simulink model "Displays_ARES_Sim"  (R2019b)
settings: Solver=FixedStepAuto  StartTime=0  StopTime=500  RelTol=1e-3  EnableMultiTasking=on
values from neighbouring files (symbols this model uses):
  Avail_Mode = 2    [Init_Vars_ARES_Sim.m]    (also in Init_Vars_ARES_Sim_SR.m = 0; Init_Vars_ARES_Sim_SR_Michael.m = 0)
  quad_s = 1    [Init_Vars_ARES_Sim.m]    (also in Init_Vars_ARES_Sim_SR.m; Init_Vars_ARES_Sim_SR_Michael.m)
  xLP0 = x0    (= 12000)    [Init_Vars_ARES_Sim.m]    (also in Init_Vars_ARES_Sim_SR.m; Init_Vars_ARES_Sim_SR_Michael.m)
  yLP0 = y0 + 1350    (= 13350)    [Init_Vars_ARES_Sim.m]    (also in Init_Vars_ARES_Sim_SR.m = 10950; Init_Vars_ARES_Sim_SR_Michael.m = 10950)
undefined symbols (not defined in the file or in its folder): LPs, var
libraries: vrlib x37, simulink x5, visionsources x3, simulink_extras x1, aerolibanimutils x1
(part 1 of 2)
settings Model: PacingRate=1.200000  Creator=DreamChaser  LastModifiedBy=ARES
settings SolverCC: AutoInsertRateTranBlk=on
settings DataIOCC: ReturnWorkspaceOutputs=off
settings DebuggingCC: MultiTaskDSMMsg=none  ArithmeticOperatorsInVariantConditions=warning
settings SFSimCC: SimUseLocalCustomCode=off  CustomCodeUndefinedFunction=UseInterfaceOnly
settings RTWCC: RTWUseLocalCustomCode=off
settings CodeAppCC: StateflowObjectComments=on

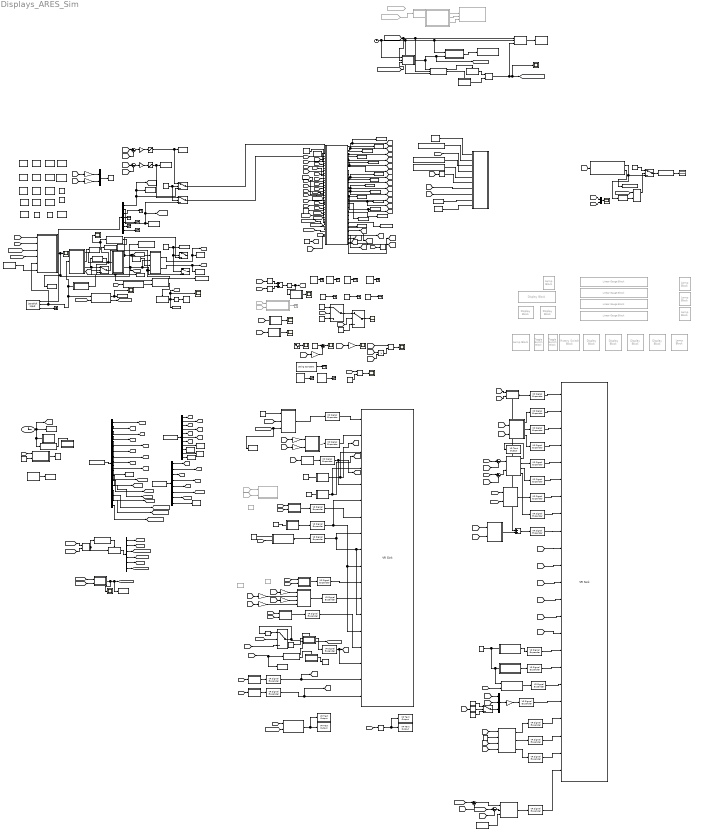
== system Displays_ARES_Sim ==
  note: Stop simulation at LP height
  note: Assure that you run initvars script
  note: Clock and Stop Condition
  note: Define Vehicle Dynamics
  note: Memory blocks intialization
  note: Input variables from Matlab
  note: Failure Modes
  note: SYSTEM DISPLAY
  note: Cache
  note: Groundspeed
  note: Heading
  note: Clearing
  note: Lunar Bat
  note: LMP Bat 2
  note: LMP Bat 1
  note: DECENT POWER
  note: COMS STATUS
  note: LANDING CONDITIONS
  note: Speed
  note: Roll
  note: Pitch
  note: LIDAR CONTROL
  note: Active
  note: Main
  note: Gain
  note: Aux
  note: Tertiary Flight Display
  note: Pitch & Roll Alarms
  note: LIDAR CONTROL
  note: COMS STATUS
  note: DECENT POWER
  note: SYSTEM DISPLAY
  note: Thrust
  note: Fuel Temp
  note: Fuel
      | Press
  note: T/W
  note: Lunar Contact
  note: Background Translation
  note: Altitude Marker
  note: Landing Site Bar
  note: Fuel bar
  note: Subject Roll Triangle
  note: Primary Flight Display (Design done in the VRSink block: assure the VRsink is open)
  note: Gudiance Cues Translation
  note: Pitch Translation Bar
  note: Background Rotation
  note: Pitch Rotation Bars
  note: Terminal Descent Bar
  note: Roll Guidance Triangle
  note: Pitch Rotation
  note: Pitch Text
  note: Autopilot 0.1
  note: HSI - Horizontal Situation Indicator
  note: Embedded Tasks
  note: Redesignation of landing sites
      | (Improvements need to be
      | made here for run speed)
  note: Workload Assessment (B&E test)
  "  2" : ToWorkspace  VariableName=abort_press  SaveFormat=Timeseries  SampleTime=-1
  "  3" : ToWorkspace  VariableName=valid_abort  SaveFormat=Timeseries  SampleTime=-1
  " 2" : ToWorkspace  VariableName=fail_detection_time  SaveFormat=Timeseries  SampleTime=-1
  " 3" : ToWorkspace  VariableName=fail_detection  SaveFormat=Timeseries  SampleTime=-1
  ASCII to String1 : ASCIIToString
  AUTO Mode Select1 : MATLAB Function  TreatAsAtomicUnit=on
  AUTO Mode Select3 : MATLAB Function  TreatAsAtomicUnit=on
  Abort_Value_Func1 : MATLAB Function  TreatAsAtomicUnit=on
  Active LIDAR : Scope
  Add : Sum
  Add1 : Sum
  Alt Triangle Pts : MATLAB Function  TreatAsAtomicUnit=on
  Aux : Terminator
  B&E function1 : MATLAB Function  TreatAsAtomicUnit=on
  B&E test1 : Display
  Background Translation : MATLAB Function  TreatAsAtomicUnit=on
  Clock : Clock
  Clock1 : Clock
  Compare To Constant : simulink/Logic and Bit Operations/Compare To Constant  relop=<=  const=250  OutDataTypeStr=boolean
  Compare To Constant1 : simulink/Logic and Bit Operations/Compare To Constant  relop=<=  const=250  OutDataTypeStr=boolean
  Constant1 : Constant  Value=Avail_Mode
  Constant11 : Constant  Value=Avail_Mode
  Constant12 : Constant  Value=3
  Constant13 : Constant  Value=100
  Constant14 : Constant  Value=260  SampleTime=-1
  Constant15 : Constant  Value=0
  Constant16 : Constant  Value=8  OutDataTypeStr=uint8
  Constant2 : Constant  Value=quad_s
  Constant22 : Constant  Value=1000
  Constant23 : Constant  Value=1.1
  Constant5 : Constant
  Constant6 : Constant
  Constant7 : Constant  Value=0
  Constant8 : Constant
  Constant9 : Constant  Value=3
  "Contact LIght " : Scope
  Data Store Memory : DataStoreMemory  DataStoreName=xLPPos  ReadBeforeWriteMsg=warning  WriteAfterWriteMsg=warning  WriteAfterReadMsg=warning  ShowAdditionalParam=off
  Data Store Memory1 : DataStoreMemory  DataStoreName=yLPPos  ReadBeforeWriteMsg=warning  WriteAfterWriteMsg=warning  WriteAfterReadMsg=warning  ShowAdditionalParam=off
  Data Store Memory10 : DataStoreMemory  DataStoreName=hTD  ReadBeforeWriteMsg=warning  WriteAfterWriteMsg=warning  WriteAfterReadMsg=warning  ShowAdditionalParam=off
  Data Store Memory11 : DataStoreMemory  DataStoreName=hLP  ReadBeforeWriteMsg=warning  WriteAfterWriteMsg=warning  WriteAfterReadMsg=warning  ShowAdditionalParam=off
  Data Store Memory12 : DataStoreMemory  DataStoreName=mp_guess  ReadBeforeWriteMsg=warning  WriteAfterWriteMsg=warning  WriteAfterReadMsg=warning  ShowAdditionalParam=off
  Data Store Memory13 : DataStoreMemory  DataStoreName=fail_type  ReadBeforeWriteMsg=warning  WriteAfterWriteMsg=warning  WriteAfterReadMsg=warning  ShowAdditionalParam=off
  Data Store Memory14 : DataStoreMemory  DataStoreName=quad_s  ReadBeforeWriteMsg=warning  WriteAfterWriteMsg=warning  WriteAfterReadMsg=warning  ShowAdditionalParam=off
  Data Store Memory17 : DataStoreMemory  DataStoreName=Mode  ReadBeforeWriteMsg=warning  WriteAfterWriteMsg=warning  WriteAfterReadMsg=warning  ShowAdditionalParam=off
  Data Store Memory19 : DataStoreMemory  DataStoreName=x_delta  ReadBeforeWriteMsg=warning  WriteAfterWriteMsg=warning  WriteAfterReadMsg=warning  ShowAdditionalParam=off
  Data Store Memory2 : DataStoreMemory  DataStoreName=xLPNeg  ReadBeforeWriteMsg=warning  WriteAfterWriteMsg=warning  WriteAfterReadMsg=warning  ShowAdditionalParam=off
  Data Store Memory20 : DataStoreMemory  DataStoreName=y_delta  ReadBeforeWriteMsg=warning  WriteAfterWriteMsg=warning  WriteAfterReadMsg=warning  ShowAdditionalParam=off
  Data Store Memory3 : DataStoreMemory  DataStoreName=yLPNeg  ReadBeforeWriteMsg=warning  WriteAfterWriteMsg=warning  WriteAfterReadMsg=warning  ShowAdditionalParam=off
  Data Store Memory4 : DataStoreMemory  DataStoreName=yLPNew  ReadBeforeWriteMsg=warning  WriteAfterWriteMsg=warning  WriteAfterReadMsg=warning  ShowAdditionalParam=off
  Data Store Memory5 : DataStoreMemory  DataStoreName=xLPNew  ReadBeforeWriteMsg=warning  WriteAfterWriteMsg=warning  WriteAfterReadMsg=warning  ShowAdditionalParam=off
  Data Store Memory6 : DataStoreMemory  DataStoreName=intervalPos  ReadBeforeWriteMsg=warning  WriteAfterWriteMsg=warning  WriteAfterReadMsg=warning  ShowAdditionalParam=off
  Data Store Memory7 : DataStoreMemory  DataStoreName=intervalNeg  ReadBeforeWriteMsg=warning  WriteAfterWriteMsg=warning  WriteAfterReadMsg=warning  ShowAdditionalParam=off
  Data Store Memory8 : DataStoreMemory  DataStoreName=interval  ReadBeforeWriteMsg=warning  WriteAfterWriteMsg=warning  WriteAfterReadMsg=warning  ShowAdditionalParam=off
  Data Store Memory9 : DataStoreMemory  DataStoreName=R0val  ReadBeforeWriteMsg=warning  WriteAfterWriteMsg=warning  WriteAfterReadMsg=warning  InitialValue=1e-12  ShowAdditionalParam=off  OutDataTypeStr=double
  Data Store Read : DataStoreRead  DataStoreName=xLPNew  SampleTime=0.1
  Data Store Read1 : DataStoreRead  DataStoreName=yLPNew  SampleTime=0.1
  Data Store Read10 : DataStoreRead  DataStoreName=hLP
  Data Store Read11 : DataStoreRead  DataStoreName=hTD
  Data Store Read12 : DataStoreRead  DataStoreName=hLP  SampleTime=0.1
  Data Store Read13 : DataStoreRead  DataStoreName=hLP  SampleTime=0.1
  Data Store Read18 : DataStoreRead  DataStoreName=hLP  SampleTime=0.1
  Data Store Read2 : DataStoreRead  DataStoreName=xLPNew
  Data Store Read21 : DataStoreRead  DataStoreName=R0val  SampleTime=0.1
  Data Store Read3 : DataStoreRead  DataStoreName=yLPNew
  Data Store Read{36..39} (4 alike) : DataStoreRead  DataStoreName=Mode
  Data Store Read6 : DataStoreRead  DataStoreName=interval
  Data Store Write12 : DataStoreWrite  DataStoreName=hTD  SampleTime=0.1
  Data Store Write13 : DataStoreWrite  DataStoreName=hLP  SampleTime=0.1
  Data Store Write14 : DataStoreWrite  DataStoreName=xLPNew  SampleTime=0.1
  Data Store Write15 : DataStoreWrite  DataStoreName=yLPNew  SampleTime=0.1
  Data Store Write20 : DataStoreWrite  DataStoreName=interval  SampleTime=0.1
  Data Store Write22 : DataStoreWrite  DataStoreName=yLPNew  SampleTime=0.1
  Data Store Write3 : DataStoreWrite  DataStoreName=Mode
  Data Store Write6 : DataStoreWrite  DataStoreName=xLPNew  SampleTime=0.1
  Data Store Write8 : DataStoreWrite  DataStoreName=R0val  SampleTime=0.1
  Define Buttons LPs1 : MATLAB Function  TreatAsAtomicUnit=on
  Delay One Step : Delay  DelayLengthSource=Input port  DelayLength=1  DelayLengthUpperLimit=3000
      settings: InputPortMap=u0,p1
  Delay1 : Delay  DelayLength=6  InitialCondition=0
  Demux : Demux  Outputs=7
  Demux2 : Demux  Outputs=6
  Demux3 : Demux  Outputs=8
  Demux6 : Demux  Outputs=11
  Demux7 : Demux  Outputs=18
  Descent Rate output : ToWorkspace  VariableName=hdot  SaveFormat=Timeseries  SampleTime=-1
  Designated Landing : MATLAB Function  TreatAsAtomicUnit=on
  Designated hTD : MATLAB Function  TreatAsAtomicUnit=on
  Detect Change5 : simulink/Logic and Bit Operations/Detect Change  vinit=0  OutDataTypeStr=boolean
  Detect Increase1 : simulink/Logic and Bit Operations/Detect Increase  vinit=0.0  OutDataTypeStr=boolean
  Detect Increase4 : simulink/Logic and Bit Operations/Detect Increase  vinit=0.0  OutDataTypeStr=boolean
  Display{1..7} (7 alike) : DisplayBlock  Commented=on  LabelPosition=Hide  Format=short  Transparency=1
  Divide : Product  Inputs=*/
  From Workspace1 : FromWorkspace  VariableName=constant_vars  SampleTime=0
  From Workspace2 : FromWorkspace  VariableName=Initial_conditions  SampleTime=0
  From Workspace5 : FromWorkspace  VariableName=input_vars  SampleTime=0
  From135 : From  Commented=on  GotoTag=fuel
  From136 : From  Commented=on  GotoTag=mdot
  From27 : From  Commented=on  GotoTag=buzz_time_1
  From29 : From  Commented=on  GotoTag=buzz_time_2
  From95 : From  Commented=on  GotoTag=VE
  From96 : From  Commented=on  GotoTag=VN
  Fuel Press : Scope
  Fuel Temp : Scope
  Gain{,2..4,6..7} (6 alike) : Gain  Gain=0.1
  Gain1 : Gain  Gain=.1
  Gain10 : Gain  Gain=20/6000
  Gain11 : Gain  Gain=1/3
  Gain12 : Gain  Gain=1/3
  Gain13 : Gain  Gain=-0.01
  Gain5 : Gain  Gain=.1
  Gain9 : Gain  Gain=100/6000
  GreaterThan3 : RelationalOperator  Operator=<=  OutDataTypeStr=boolean  RndMeth=Simplest
  Groundspeed : MATLAB Function  TreatAsAtomicUnit=on
  Guidance Cross : MATLAB Function  TreatAsAtomicUnit=on
  Guidance Triangle : MATLAB Function  TreatAsAtomicUnit=on
  HSD_model : ModelReference  ModelNameDialog=HSD_model  SimulationMode=Normal  ModelReferenceVersion=1.1662
  HSI_Acc1 : MATLAB Function  TreatAsAtomicUnit=on
  HSI_Ball : MATLAB Function  TreatAsAtomicUnit=on
  HSI_LP : MATLAB Function  TreatAsAtomicUnit=on
  HSI_VG : MATLAB Function  TreatAsAtomicUnit=on
  HSI_Vec : MATLAB Function  TreatAsAtomicUnit=on
  Heading : Terminator  Commented=on
  IPC Mode Select2 : MATLAB Function  TreatAsAtomicUnit=on
  If : If  ElseIfExpressions=u1<0  ShowElse=off
  If Action Subsystem : Subsystem  TreatAsAtomicUnit=on
  If Action Subsystem1 : Subsystem  TreatAsAtomicUnit=on
  If Action Subsystem2 : Subsystem  TreatAsAtomicUnit=on
  If Action Subsystem3 : Subsystem  TreatAsAtomicUnit=on
  If Action Subsystem5 : Subsystem  TreatAsAtomicUnit=on
  If Action Subsystem6 : Subsystem  TreatAsAtomicUnit=on
  If Action Subsystem7 : Subsystem  TreatAsAtomicUnit=on
  If Action Subsystem8 : Subsystem  TreatAsAtomicUnit=on
  If Action Subsystem9 : Subsystem  TreatAsAtomicUnit=on
  If1 : If  NumInputs=3  IfExpression=u1==1  ElseIfExpressions=u2==u3
  If2 : If  IfExpression=u1 ~= 0  ShowElse=off
  If4 : If  ShowElse=off
  If5 : If  IfExpression=u1 ~= 0  ShowElse=off
  If6 : If  IfExpression=u1 < 0.0003  ShowElse=off
  If9 : If  NumInputs=2  IfExpression=u1 ==1 & u2 ==1  ShowElse=off
  Image From File7 : visionsources/Image From File  Tag=vipblks_nd  FileName=C:\Users\ARES\Documents\ARES Simulation SR\Graphics\Abort_Photo_V1.jpg  Ts=-1  imagePorts=One multidimensional signal  OutPortLabels=R|G|B  ImageDataType=int32  sdImageDataType=uint(8)  Signed=on  WordLength=16  FractionLengthMode=User-defined  FractionLength=15
      settings: SourceProductName=Computer Vision Toolbox
  Image From File8 : visionsources/Image From File  Tag=vipblks_nd  FileName=C:\Users\ARES\Documents\ARES Simulation SR\ALD_Map_Hazzards.png  Ts=-1  imagePorts=One multidimensional signal  OutPortLabels=R|G|B  ImageDataType=int32  sdImageDataType=uint(8)  Signed=on  WordLength=16  FractionLengthMode=User-defined  FractionLength=15
      settings: SourceProductName=Computer Vision Toolbox
  Image From File9 : visionsources/Image From File  Tag=vipblks_nd  FileName=C:\Users\ARES\Documents\ARES Simulation SR\ALD_Map_No_Hazzards.png  Ts=-1  imagePorts=One multidimensional signal  OutPortLabels=R|G|B  ImageDataType=int32  sdImageDataType=uint(8)  Signed=on  WordLength=16  FractionLengthMode=User-defined  FractionLength=15
      settings: SourceProductName=Computer Vision Toolbox
  Joystick Input2 : vrlib/Joystick Input  joyid=1  adjustports=on  forcefeed=off
      settings: SourceProductBaseCode=VR
  LMP 1 : Terminator
  LMP 2 : Terminator
  Lamp{,1..5} (6 alike) : LampBlock  Commented=on  LabelPosition=Hide
  Lidar Gain : Terminator
  Linear Gauge : LinearGaugeBlock  Commented=on  LabelPosition=Hide  TickInterval=20
  Linear Gauge1 : LinearGaugeBlock  Commented=on  LabelPosition=Hide  ScaleMin=40  TickInterval=10
  Linear Gauge2 : LinearGaugeBlock  Commented=on  LabelPosition=Hide  ScaleMax=6  TickInterval=1
  Linear Gauge3 : LinearGaugeBlock  Commented=on  LabelPosition=Hide  ScaleMax=300  TickInterval=50
  Lunar Bat : Terminator
  MA : Terminator
  MATLAB Function : MATLAB Function  Commented=on  TreatAsAtomicUnit=on
  MATLAB Function1 : MATLAB Function  TreatAsAtomicUnit=on
  MATLAB Function10 : MATLAB Function  Commented=on  TreatAsAtomicUnit=on
  MATLAB Function11 : MATLAB Function  TreatAsAtomicUnit=on
  MATLAB Function12 : MATLAB Function  TreatAsAtomicUnit=on
  MATLAB Function13 : MATLAB Function  TreatAsAtomicUnit=on
  MATLAB Function14 : MATLAB Function  TreatAsAtomicUnit=on
  MATLAB Function15 : MATLAB Function  TreatAsAtomicUnit=on
  MATLAB Function16 : MATLAB Function  TreatAsAtomicUnit=on
  MATLAB Function17 : MATLAB Function  TreatAsAtomicUnit=on
  MATLAB Function18 : MATLAB Function  TreatAsAtomicUnit=on
  MATLAB Function2 : MATLAB Function  TreatAsAtomicUnit=on
  MATLAB Function3 : MATLAB Function  Commented=on  TreatAsAtomicUnit=on
  MATLAB Function4 : MATLAB Function  Commented=on  TreatAsAtomicUnit=on
  MATLAB Function5 : MATLAB Function  TreatAsAtomicUnit=on
  MATLAB Function6 : MATLAB Function  TreatAsAtomicUnit=on
  MATLAB Function7 : MATLAB Function  Commented=on  TreatAsAtomicUnit=on
  MATLAB Function8 : MATLAB Function  TreatAsAtomicUnit=on
  MATLAB Function9 : MATLAB Function  TreatAsAtomicUnit=on
  Main : Terminator
  Memory : Memory
  Merge : Merge
  Mux : Mux  Inputs=2
  Mux3 : Mux  Inputs=3
  Mux4 : Mux  Inputs=2
  Overpitch Scope : Scope
  Overroll Scope : Scope
  Overspeed Scope : Scope
  Pitch & Roll1 : Scope
  Pitch Translation Bars : MATLAB Function  TreatAsAtomicUnit=on
  Pitch TranslationText : MATLAB Function  TreatAsAtomicUnit=on
  Product : Product
  Pulse Generator : DiscretePulseGenerator  PulseType=Time based  Period=1/6  PulseWidth=50
  RCAH Mode Select1 : MATLAB Function  TreatAsAtomicUnit=on
  Roll Triangle : MATLAB Function  TreatAsAtomicUnit=on
  Rotary Switch : RotarySwitchBlock  Commented=on  LabelPosition=Hide
      settings: Values={{'Off', 'Low', 'Medium', 'High'}, [0 1 2 3]}
  Rotations : MATLAB Function  TreatAsAtomicUnit=on
  Round : Rounding  Operator=round
  S-R Flip-Flop1 : simulink_extras/Flip Flops/S-R Flip-Flop  initial_condition=0
  Saturation : Saturate  UpperLimit=1  LowerLimit=-1
  Saturation1 : Saturate  UpperLimit=1  LowerLimit=-1
  Scope{,1..5} (6 alike) : Scope
  Secondary Workload : MATLAB Function  TreatAsAtomicUnit=on
  Simulation Pace : aerolibanimutils/Simulation Pace  SimulationPace=1  SleepMode=MATLAB Thread  OutputPaceError=off  SampleTime=1/30
  Sine Wave : Sin  Amplitude=2  Bias=70  Frequency=2*pi/120  SampleTime=0
  Sqrt : Sqrt  SaturateOnIntegerOverflow=on
  Square : Math  Operator=square  SignedPower=off  SaturateOnIntegerOverflow=on
  Square1 : Math  Operator=square  SignedPower=off  SaturateOnIntegerOverflow=on
  Stop Simulation2 : Stop
  Stop Simulation3 : Stop
  Stop Simulation4 : Stop
  String Constant1 : StringConstant  String="\"29 V\""
  String Constant2 : StringConstant  String="\"30 V\""
  String Constant3 : StringConstant  String="\"32 V\""
  String Constant4 : StringConstant  String="\"AQ\""
  String Constant5 : StringConstant  String="\"MASTER ALARM\""
  String Constant6 : StringConstant  String="\"TEMP\""
  String Constant7 : StringConstant  String="\"NO ATT\""
  Subsystem1 : Subsystem
  Sum{,1..2,4..7} (7 alike) : Sum  Inputs=|+-
  Switch{,7..8,10..12} (6 alike) : Switch  Criteria=u2 > Threshold
  Switch2 : Switch  Criteria=u2 > Threshold  Threshold=1
  Switch3 : Switch  Criteria=u2 > Threshold  Threshold=250
  Switch4 : Switch  Criteria=u2 > Threshold  Threshold=225
  Switch5 : Switch  Criteria=u2 > Threshold  Threshold=1
  T/W : Scope
  "TA " : Terminator
  TA 1 : Terminator
  Terminator{,1..4,6} (6 alike) : Terminator
  Thrust : Scope
  To Workspace : ToWorkspace  VariableName=R  SaveFormat=Timeseries  SampleTime=-1
  To Workspace1 : ToWorkspace  VariableName=thetaG  SaveFormat=Timeseries  SampleTime=-1
  To Workspace10 : ToWorkspace  VariableName=LP_button  SaveFormat=Timeseries  SampleTime=-1
  To Workspace11 : ToWorkspace  VariableName=IPC_button  SaveFormat=Timeseries  SampleTime=-1
  To Workspace13 : ToWorkspace  VariableName=roll_gain_fail  SaveFormat=Timeseries  SampleTime=-1
  To Workspace14 : ToWorkspace  VariableName=pitch_gain_fail  SaveFormat=Timeseries  SampleTime=-1
  To Workspace15 : ToWorkspace  VariableName=reversal_fail  SaveFormat=Timeseries  SampleTime=-1
  To Workspace16 : ToWorkspace  VariableName=stuck_fail  SaveFormat=Timeseries  SampleTime=-1
  To Workspace17 : ToWorkspace  VariableName=fail_percent  SaveFormat=Timeseries  SampleTime=-1
  To Workspace18 : ToWorkspace  VariableName=RealTime  SampleTime=-1
  To Workspace19 : ToWorkspace  VariableName=fail_roll_triangle  SaveFormat=Timeseries  SampleTime=-1
  To Workspace2 : ToWorkspace  VariableName=phiG  SaveFormat=Timeseries  SampleTime=-1
  To Workspace20 : ToWorkspace  VariableName=fuel_fail_out  SaveFormat=Timeseries  SampleTime=-1
  To Workspace24 : ToWorkspace  VariableName=pitch_comm1  SaveFormat=Timeseries  SampleTime=-1
  To Workspace25 : ToWorkspace  VariableName=roll_comm1  SaveFormat=Timeseries  SampleTime=-1
  To Workspace3 : ToWorkspace  VariableName=Time  SaveFormat=Timeseries  SampleTime=-1
  To Workspace4 : ToWorkspace  VariableName=fuel  SaveFormat=Timeseries  SampleTime=-1
  To Workspace5 : ToWorkspace  VariableName=pitch_comm  SaveFormat=Timeseries  SampleTime=-1
  To Workspace6 : ToWorkspace  VariableName=roll_comm  SaveFormat=Timeseries  SampleTime=-1
  To Workspace7 : ToWorkspace  VariableName=Auditory_TIME_BUTTON  SaveFormat=Timeseries  SampleTime=-1
      settings: Save2DSignal=2-D array (concatenate along first dimension)
  Toggle Switch : ToggleSwitchBlock  Commented=on  LabelPosition=Hide
      settings: Values={{'Off', 'On'}, [0 1]}
  Toggle Switch1 : ToggleSwitchBlock  Commented=on  LabelPosition=Hide
      settings: Values={{'Off', 'On'}, [0 1]}
  Uplink : Terminator
  VE output : ToWorkspace  VariableName=VE  SaveFormat=Timeseries  SampleTime=-1
      settings: Save2DSignal=2-D array (concatenate along first dimension)
  VN output : ToWorkspace  VariableName=VN  SaveFormat=Timeseries  SampleTime=-1
  VN output2 : ToWorkspace  VariableName=Mode  SaveFormat=Timeseries  SampleTime=-1
  VR Signal Expander : vrlib/VR Signal Expander  outwidth=3  outidx=[1,2,3]
      settings: SourceProductName=Simulink 3D Animation  SourceProductBaseCode=VR
  VR Signal Expander1 : vrlib/VR Signal Expander  outwidth=3  outidx=[1,2,3]
      settings: SourceProductName=Simulink 3D Animation  SourceProductBaseCode=VR
  VR Signal Expander10 : vrlib/VR Signal Expander  outwidth=3  outidx=[2]
      settings: SourceProductName=Simulink 3D Animation  SourceProductBaseCode=VR
  VR Signal Expander{5,8,11,23,33..36} (8 alike) : vrlib/VR Signal Expander  outwidth=3  outidx=[1 2 3]
      VR Signal Expander11 settings: SourceProductName=Simulink
      VR Signal Expander23 settings: SourceProductName=Simulink
      VR Signal Expander33 settings: SourceProductName=Simulink
      VR Signal Expander34 settings: SourceProductName=Simulink
      VR Signal Expander35 settings: SourceProductName=Simulink
      VR Signal Expander36 settings: SourceProductName=Simulink
      VR Signal Expander5 settings: SourceProductName=Simulink 3D Animation  SourceProductBaseCode=VR
      VR Signal Expander8 settings: SourceProductName=Simulink 3D Animation  SourceProductBaseCode=VR
  VR Signal Expander{2,6..7,12..13,17,30..32} (9 alike) : vrlib/VR Signal Expander  outwidth=3  outidx=[1 2]
      VR Signal Expander12 settings: SourceProductName=Simulink
      VR Signal Expander13 settings: SourceProductName=Simulink
      VR Signal Expander17 settings: SourceProductName=Simulink
      VR Signal Expander2 settings: SourceProductName=Simulink 3D Animation  SourceProductBaseCode=VR
      VR Signal Expander30 settings: SourceProductName=Simulink
      VR Signal Expander31 settings: SourceProductName=Simulink
      VR Signal Expander32 settings: SourceProductName=Simulink
      VR Signal Expander6 settings: SourceProductName=Simulink 3D Animation  SourceProductBaseCode=VR
      VR Signal Expander7 settings: SourceProductName=Simulink 3D Animation  SourceProductBaseCode=VR
  VR Signal Expander14 : vrlib/VR Signal Expander  outwidth=4  outidx=[4]
      settings: SourceProductName=Simulink
  VR Signal Expander15 : vrlib/VR Signal Expander  outwidth=3  outidx=[2]
      settings: SourceProductName=Simulink
  VR Signal Expander16 : vrlib/VR Signal Expander  outwidth=4  outidx=[4]
      settings: SourceProductName=Simulink
  VR Signal Expander18 : vrlib/VR Signal Expander  outwidth=3  outidx=[3]
      settings: SourceProductName=Simulink
  VR Signal Expander19 : vrlib/VR Signal Expander  outwidth=3  outidx=[3]
      settings: SourceProductName=Simulink
  VR Signal Expander20 : vrlib/VR Signal Expander  outwidth=3  outidx=[3]
      settings: SourceProductName=Simulink
  VR Signal Expander3 : vrlib/VR Signal Expander  outwidth=4  outidx=[3 4]
      settings: SourceProductName=Simulink 3D Animation  SourceProductBaseCode=VR
  VR Signal Expander4 : vrlib/VR Signal Expander  outwidth=3  outidx=[1,2]
      settings: SourceProductName=Simulink 3D Animation  SourceProductBaseCode=VR
  VR Signal Expander9 : vrlib/VR Signal Expander  outwidth=3  outidx=[1,2,3]
      settings: SourceProductName=Simulink 3D Animation  SourceProductBaseCode=VR
  VR Sink : vrlib/VR Sink  InstantiateOnLoad=on  SampleTime=0.1  ViewEnable=on  RemoteChange=off  RemoteView=off  FieldsWritten=Vel_Ball.translation.3.1.1.double#Vel_Vector.rotation.4.1.1.double#Vel_Vector.scale.3.1.1.double#Vel_Vector.translation.3.1.1.double#Guide_Heading_Rot.rotation.4.1.1.double#LP.translation.3.1.1.double#Guidance_Velocity.translation.3.1.1.double#Landing_Point.translation.3.1.1.double#Ship_accel.translation.3.1.1.double#FuelGauge.scale.3.1.1.double#DesignatedLanding.translation.3.1.1.double#DesignatedHTD.translation.3.1.1.double#AltitudeTriangle.translation.3.1.1.double#AltitudeTriangle_0002.translation.3.1.1.double#AltitudeTriangle_0001.translation.3.1.1.double#RCAH_Color.diffuseColor.3.1.1.double#IPC_Color.diffuseColor.3.1.1.double#AUTO_Color.diffuseColor.3.1.1.double#Map.translation.3.1.1.double#Abort.translation.3.1.1.double#Land.translation.3.1.1.double#Fuel_img.translation.3.1.1.double#Original_LP.translation.3.1.1.double  WorldFileName=VRWorlds\hsi.wrl  AutoView=on  VideoDimensions=[]  AllowVariableSize=off  FigureProperties="{'Position', 'Name', 'Viewpoint', 'CameraBound', 'CameraDirection', 'CameraPosition', 'CameraUpVector', 'ZoomFactor', 'Antialiasing', 'Headlight', 'Lighting', 'NavPanel', 'Sound', 'StatusBar', 'Stereo3D', 'Stereo3DCameraOffset', 'Stereo3DHIT', 'ToolBar', 'Textures', 'Transparency', 'Triad', 'Wireframe', 'NavZones', 'NavMode', 'NavSpeed', 'CaptureFileFormat', 'CaptureFileName', 'Record2DCompressMethod', 'Record2DCompressQuality', 'Record2D', 'Record2DFileName', 'Record2DFPS'; [-1.0240000000000000e+03   7.2500000000000000e+02   1.0200000000000000e+03   5.0200000000000000e+02], '', '_untitled_1', 'on', [7.1821279555918119e-02  -7.1914500889074973e-02  -9.9482159624971234e-01], [0.0000000000000000e+00   0.0000000000000000e+00   0.0000000000000000e+00], [3.8829635941558640e-03   9.9740995904225715e-01  -7.1821279555918133e-02], [1.0000000000000000e+00], 'on', 'on', 'on', 'halfbar', 'on', 'on', 'off', [1.0000000149011612e-01], [0.0000000000000000e+00], 'on', 'on', 'on', 'none', 'off', 'off', 'fly', 'normal', 'tif', '%f_anim_%n.tif', 'auto', [7.5000000000000000e+01], 'off', '%f_anim_%n.avi', 'auto'}"
      settings: SourceProductName=Simulink
  VR Sink1 : vrlib/VR Sink  InstantiateOnLoad=on  SampleTime=0.1  ViewEnable=on  RemoteChange=off  RemoteView=off  FieldsWritten=BotTriangle.translation.3.1.1.double#TopTriangle.translation.3.1.1.double#DesignatedLanding.translation.3.1.1.double#DesignatedHTD.translation.3.1.1.double#AltitudeTriangle.translation.3.1.1.double#Rotating.rotation.4.1.1.double#Rotating.translation.3.1.1.double#Right_bar.diffuseColor.3.1.1.double#LeftPitch.diffuseColor.3.1.1.double#PitchText.rotation.4.1.1.double#PitchText.translation.3.1.1.double#Cross.translation.3.1.1.double#Piper.diffuseColor.3.1.1.double#BotBack.rotation.4.1.1.double#BotBack.translation.3.1.1.double#FuelGauge.scale.3.1.1.double#AltitudeTriangle_0001.translation.3.1.1.double#AltitudeTriangle_0002.translation.3.1.1.double  WorldFileName=VRWorlds\VRWorld1.wrl  AutoView=on  VideoDimensions=[]  AllowVariableSize=off  FigureProperties="{'Position', 'Name', 'Viewpoint', 'CameraBound', 'CameraDirection', 'CameraPosition', 'CameraUpVector', 'ZoomFactor', 'Antialiasing', 'Headlight', 'Lighting', 'NavPanel', 'Sound', 'StatusBar', 'Stereo3D', 'Stereo3DCameraOffset', 'Stereo3DHIT', 'ToolBar', 'Textures', 'Transparency', 'Triad', 'Wireframe', 'NavZones', 'NavMode', 'NavSpeed', 'CaptureFileFormat', 'CaptureFileName', 'Record2DCompressMethod', 'Record2DCompressQuality', 'Record2D', 'Record2DFileName', 'Record2DFPS'; [-1.0180000000000000e+03   7.3000000000000000e+01   1.0080000000000000e+03   5.8200000000000000e+02], '', 'View', 'on', [3.1395253498715962e-02  -3.1410752802896694e-02  -9.9901336460835521e-01], [0.0000000000000000e+00   0.0000000000000000e+00   0.0000000000000000e+00], [9.8663539164468286e-04   9.9950656056293863e-01  -3.1395253498715962e-02], [1.0000000000000000e+00], 'on', 'on', 'on', 'halfbar', 'on', 'off', 'off', [1.0000000149011612e-01], [0.0000000000000000e+00], 'off', 'on', 'on', 'none', 'off', 'off', 'fly', 'normal', 'tif', '%f_anim_%n.tif', 'auto', [7.5000000000000000e+01], 'off', '%f_anim_%n.avi', 'auto'}"
      settings: SourceProductBaseCode=VR
  VR Text Output : vrlib/VR Text Output  VrmlFile=C:\Users\ARES\Documents\ARES Simulation SR\VRWorlds\VRWorld1.wrl  TxtNode=sec2emp  FormatString=%d  Ts=-1  ForceViewerOpen=off
      settings: SourceProductName=Simulink  SourceProductBaseCode=SL
  VR Text Output1 : vrlib/VR Text Output  VrmlFile=C:\Users\ARES\Documents\ARES Simulation SR\VRWorlds\hsi.wrl  TxtNode=sec2emp  FormatString=%d  Ts=-1  ForceViewerOpen=off
      settings: SourceProductName=Simulink  SourceProductBaseCode=SL
  VR Text Output2 : vrlib/VR Text Output  VrmlFile=C:\Users\ARES\Documents\ARES Acheivability Limit Research\Simulink Models\ALA and Controls Experiment\VR Worlds\hsi.wrl  TxtNode=Range_txt  FormatString=%d  Ts=-1  ForceViewerOpen=off
      settings: SourceProductName=Simulink  SourceProductBaseCode=SL
  VR Text Output3 : vrlib/VR Text Output  VrmlFile=C:\Users\ARES\Documents\ARES Simulation SR\VRWorlds\VRWorld1.wrl  TxtNode=gs_digital  FormatString=%d  Ts=-1  ForceViewerOpen=off
      settings: SourceProductName=Simulink  SourceProductBaseCode=SL
  VR Text Output4 : vrlib/VR Text Output  VrmlFile=C:\Users\ARES\Documents\ARES Simulation SR\VRWorlds\hsi.wrl  TxtNode=gs_digital  FormatString=%d  Ts=-1  ForceViewerOpen=off
      settings: SourceProductName=Simulink  SourceProductBaseCode=SL
  "Vehicle Dynamics " : Subsystem
  Vertical Rate : MATLAB Function  TreatAsAtomicUnit=on
  XY Memory : DataStoreMemory  DataStoreName=XY  ReadBeforeWriteMsg=warning  WriteAfterWriteMsg=warning  WriteAfterReadMsg=warning  InitialValue=[500 500]  VectorParams1D=off  ShowAdditionalParam=off
  XY Imaging Input : DataStoreRead  Commented=on  DataStoreName=XY  DataStoreElements=XY
  XY Imaging Input2 : DataStoreRead  DataStoreName=XY  DataStoreElements=XY
  XY Imaging Input3 : DataStoreRead  DataStoreName=XY  DataStoreElements=XY
  XY Imaging Input5 : DataStoreRead  Commented=on  DataStoreName=XY  DataStoreElements=XY
  XY Imaging Input6 : DataStoreRead  Commented=on  DataStoreName=XY  DataStoreElements=XY
  XY Storage : DataStoreWrite  DataStoreName=XY  SampleTime=0.1  DataStoreElements=XY
  h output : ToWorkspace  VariableName=h  SaveFormat=Timeseries  SampleTime=-1
  mp_guess : DataStoreWrite  DataStoreName=mp_guess  SampleTime=0.1
  pitch output : ToWorkspace  VariableName=pitch  SaveFormat=Timeseries  SampleTime=-1
  roll angle output : ToWorkspace  VariableName=roll  SaveFormat=Timeseries  SampleTime=-1
  time_to_empty : MATLAB Function  TreatAsAtomicUnit=on
  xpos output : ToWorkspace  VariableName=xpos  SaveFormat=Timeseries  SampleTime=-1
  ypos output : ToWorkspace  VariableName=ypos  SaveFormat=Timeseries  SampleTime=-1
  wires:
  Demux/1 -> Switch2/3, [roll_comm], To Workspace6/1
  Demux/2 -> To Workspace5/1, [pitch_comm], Switch5/3
  Demux/3 -> Terminator/1
  Demux/4 -> Terminator1/1
  Demux/5 -> Terminator2/1
  Demux/6 -> Terminator3/1
  Demux/7 -> Terminator4/1
  "Vehicle Dynamics "/1(roll angle) -> roll angle output/1, [phi]
  [phi0] -> "Vehicle Dynamics "/5(phi0)
  [VE0] -> "Vehicle Dynamics "/6(VE0)
  [y0] -> "Vehicle Dynamics "/7(y0)
  [theta0] -> "Vehicle Dynamics "/8("theta0 ")
  [VN0] -> "Vehicle Dynamics "/9(VN0)
  [x0] -> "Vehicle Dynamics "/10("x0 ")
  [hdot0] -> "Vehicle Dynamics "/11(hdot0)
  [h0] -> "Vehicle Dynamics "/12(h0)
  [m_fuel0] -> "Vehicle Dynamics "/13(m_fuel)
  [R0] -> "Vehicle Dynamics "/14(R0)
  [gBody] -> "Vehicle Dynamics "/16(gBody)
  [tauV] -> "Vehicle Dynamics "/17(tauV)
  [tauT] -> "Vehicle Dynamics "/18(tauT)
  [tauh] -> "Vehicle Dynamics "/19(tauh)
  [g0] -> "Vehicle Dynamics "/20(g0)
  [Isp] -> "Vehicle Dynamics "/21(Isp)
  [m_Lander] -> "Vehicle Dynamics "/22(m_lander)
  Mux/1 -> XY Storage/1
  "Vehicle Dynamics "/7(fuel) -> To Workspace4/1, [fuel]
  Gain/1 -> Mux/1
  Gain1/1 -> Mux/2
  "Vehicle Dynamics "/5(h) -> h output/1, [h]
  "Vehicle Dynamics "/3(xpos) -> [xpos], xpos output/1
  "Vehicle Dynamics "/4("ypos ") -> [ypos], ypos output/1
  "Vehicle Dynamics "/8(phiG) -> [phiG], To Workspace2/1
  "Vehicle Dynamics "/9(thetaG) -> To Workspace1/1, [thetaG]
  [phi] -> Gain/1
  [theta] -> Gain1/1
  "Vehicle Dynamics "/6(m) -> [m]
  "Vehicle Dynamics "/10(VE) -> VE output/1, [VE]
  "Vehicle Dynamics "/11(VN) -> [VN], VN output/1
  "Vehicle Dynamics "/12("hdot ") -> [hdot], Descent Rate output/1
  [a] -> "Vehicle Dynamics "/15(a)
  Data Store Read12/1 -> "Vehicle Dynamics "/27(hLP)
  [q] -> "Vehicle Dynamics "/26(q)
  [b] -> "Vehicle Dynamics "/23("b ")
  [C] -> "Vehicle Dynamics "/24(C)
  [k] -> "Vehicle Dynamics "/25(k)
  [h] -> Subsystem1/1(h)
  Data Store Read13/1 -> Subsystem1/2(hLP)
  "Vehicle Dynamics "/13(R) -> To Workspace/1, [R]
  Clock/1 -> If6/1, MATLAB Function1/1(Time), To Workspace3/1, [Time]
  From Workspace2/1 -> Demux7/1
  Demux7/1 -> [m_fuel0]
  Demux7/2 -> [x0]
  Demux7/3 -> [y0]
  Demux7/4 -> [VE0]
  Demux7/5 -> [VN0]
  Demux7/6 -> [theta0]
  Demux7/7 -> [phi0]
  Demux7/8 -> [h0]
  From Workspace5/1 -> Demux6/1
  Demux6/3 -> [a]
  Demux6/4 -> [b]
  Demux6/5 -> [C]
  Demux6/6 -> [k]
  Demux6/7 -> [q]
  Demux6/8 -> Data Store Write14/1
  Demux6/9 -> Data Store Write15/1
  Demux7/9 -> [hdot0]
  Demux6/10 -> Data Store Write12/1
  Demux6/11 -> Data Store Write13/1
  Demux6/2 -> [gBody]
  Demux6/1 -> [R0]
  From Workspace1/1 -> Demux3/1
  Demux3/1 -> [tauV]
  Demux3/3 -> [tauh]
  Demux3/2 -> [tauT]
  Demux3/4 -> [g0]
  Demux3/5 -> [Isp]
  Demux3/6 -> [m_Lander]
  Demux3/7 -> [R_R0_tol]
  [R_R0_tol] -> "Vehicle Dynamics "/28(R_R0_tol)
  Data Store Read/1 -> "Vehicle Dynamics "/3(xLP)
  Data Store Read1/1 -> "Vehicle Dynamics "/4(yLP)
  "Vehicle Dynamics "/14(roll_gain_fail) -> To Workspace13/1
  "Vehicle Dynamics "/15(pitch_gain_fail) -> To Workspace14/1
  If Action Subsystem5/1(Out1) -> Demux2/1
  If4/1 -> If Action Subsystem5/Action
  Delay One Step/1 -> If4/1, If Action Subsystem5/1(In1)
  [fail_type] -> Delay One Step/1
  [fail_time] -> Delay One Step/2
  Demux2/1 -> [pitch_fail]
  Demux2/2 -> [roll_fail]
  Demux2/3 -> [control_reversal]
  Demux2/4 -> [thruster_fail]
  [roll_fail] -> "Vehicle Dynamics "/29(roll_fail)
  [pitch_fail] -> "Vehicle Dynamics "/30(pitch_fail)
  [control_reversal] -> "Vehicle Dynamics "/31(control_reversal)
  "Vehicle Dynamics "/16(reversal_fail) -> To Workspace15/1
  [thruster_fail] -> "Vehicle Dynamics "/32(thruster_fail)
  "Vehicle Dynamics "/17(stuck_fail) -> To Workspace16/1
  Demux2/5 -> [fuel_fail]
  [fail_time_s] -> MATLAB Function2/2(s)
  [gradual_val] -> "Vehicle Dynamics "/33(gradual_val)
  MATLAB Function2/1(y) -> Scope/1, To Workspace17/1, [gradual_val]
  [Time] -> MATLAB Function2/1(u)
  "Vehicle Dynamics "/18(hG) -> [hG]
  "Vehicle Dynamics "/19("vng ") -> [VNG]
  "Vehicle Dynamics "/20(veg) -> [VEG]
  Demux7/10 -> mp_guess/1
  Demux7/11 -> [fail_type]
  Demux7/12 -> [fail_time]
  Demux7/13 -> [fail_time_s]
  Demux7/14 -> [fail_detect]
  MATLAB Function5/1(t) -> To Workspace18/1
  If6/1 -> If Action Subsystem8/Action
  Demux2/6 -> [rolltriangle_fail]
  Demux7/15 -> [quad_s]
  Subsystem1/1(STOP) -> Stop Simulation2/1
  [VN] -> Square/1
  [VE] -> Square1/1
  Square1/1 -> Add/1
  Square/1 -> Add/2
  Add/1 -> Sqrt/1
  Sqrt/1 -> MATLAB Function13/1(theta), [Speed]
  From96/1 -> MATLAB Function4/2(VN)
  From95/1 -> MATLAB Function4/1(VE)
  MATLAB Function4/1(heading) -> Heading/1
  MATLAB Function13/1(y) -> Overspeed Scope/1
  MATLAB Function11/1(y) -> Overpitch Scope/1
  MATLAB Function12/1(y) -> Overroll Scope/1
  Constant5/1 -> Lidar Gain/1
  Constant6/1 -> Main/1
  Constant7/1 -> Aux/1
  [h] -> Switch3/2
  Constant8/1 -> Switch3/1
  Pulse Generator/1 -> Switch3/3
  Switch3/1 -> Switch4/1
  Switch4/1 -> Active LIDAR/1
  [h] -> Switch4/2
  Constant9/1 -> Switch4/3
  String Constant1/1 -> LMP 1/1
  String Constant2/1 -> LMP 2/1
  String Constant3/1 -> Lunar Bat/1
  String Constant4/1 -> Uplink/1
  [phi] -> MATLAB Function12/1(theta)
  [theta] -> MATLAB Function11/1(theta)
  "Vehicle Dynamics "/21(Thrust) -> [Thrust]
  [Thrust] -> Gain9/1
  Gain9/1 -> Thrust/1
  [m] -> Product/1
  [gBody] -> Product/2
  [Thrust] -> Divide/1
  Product/1 -> Divide/2
  Divide/1 -> T/W/1
  Sine Wave/1 -> Fuel Temp/1
  Gain10/1 -> Sum2/2
  [Thrust] -> Gain10/1
  Constant14/1 -> Sum2/1
  Sum2/1 -> Fuel Press/1
  String Constant5/1 -> MA/1
  Constant12/1 -> GreaterThan3/2
  GreaterThan3/1 -> "Contact LIght "/1
  [h] -> GreaterThan3/1
  String Constant6/1 -> "TA "/1
  String Constant7/1 -> TA 1/1
  "Vehicle Dynamics "/22(mdot) -> [mdot]
  Data Store Read21/1 -> [R0val_var]
  [R0val_var] -> "Vehicle Dynamics "/34(R0val1)
  "Vehicle Dynamics "/23(R0val2) -> [R0val_var_out]
  [R0val_var] -> Data Store Write8/1
  Alt Triangle Pts/1(pts) -> VR Signal Expander2/1
  Guidance Cross/1(pts) -> VR Signal Expander5/1
  Background Translation/1(pts) -> VR Signal Expander/1
  [theta] -> Gain5/1
  Gain3/1 -> Guidance Cross/2(phiG)
  Gain4/1 -> Guidance Cross/4(phi)
  [phiG] -> Gain3/1
  [thetaG] -> Gain2/1
  Gain6/1 -> Guidance Triangle/2(phi)
  [phiG] -> Gain7/1
  Gain7/1 -> Guidance Triangle/1(phiG)
  [phi] -> Gain6/1
  Guidance Triangle/1(pts) -> VR Signal Expander8/1
  [h] -> Alt Triangle Pts/1(h)
  VR Signal Expander9/1 -> VR Sink1/17, [at1_t]
  Designated hTD/1(pts) -> VR Sink1/4, [dhtd_t]
  Designated Landing/1(pts) -> VR Sink1/3, [dl_t]
  [m] -> time_to_empty/1(m)
  time_to_empty/1(tte) -> VR Text Output1/1, VR Text Output/1  "time_to_empty"
  [phi] -> Background Translation/2(roll)
  [theta] -> Background Translation/1(pitch)
  Data Store Read11/1 -> Designated hTD/1(height_hTD)
  If/1 -> If Action Subsystem/Action
  [fuel] -> Switch/3
  Data Store Read10/1 -> Designated Landing/1(heightLP)
  [m_Lander] -> time_to_empty/2(m_Lander)
  [theta] -> Pitch TranslationText/1(pitch)
  [phi] -> Pitch TranslationText/2(roll)
  From135/1 -> MATLAB Function3/2(fuel)
  Rotations/1(pts) -> VR Signal Expander3/1
  From136/1 -> MATLAB Function3/1(mdot)
  [Speed] -> Groundspeed/1(v)
  XY Imaging Input2/1 -> Rotations/1(xy)
  [gradual_val] -> Roll Triangle/2(gradual)
  XY Imaging Input3/1 -> Roll Triangle/1(xy)
  [theta] -> Pitch Translation Bars/1(pitch)
  [rolltriangle_fail] -> To Workspace19/1, Roll Triangle/3(fail)
  Groundspeed/1(y) -> VR Signal Expander9/1
  If Action Subsystem/2(fuel%) -> [fuel_percent]
  If/2 -> If Action Subsystem1/Action
  Pitch Translation Bars/1(pts) -> VR Signal Expander6/1
  If Action Subsystem/1(pts) -> VR Signal Expander1/1
  Memory/1 -> Switch/1
  Switch/1 -> If Action Subsystem/1(fuel), Memory/1
  VR Signal Expander2/1 -> VR Sink1/5, [at_t]
  Gain2/1 -> Guidance Cross/1(thetaG)
  Constant13/1 -> If Action Subsystem/2(m_fuel0)
  Vertical Rate/1(y) -> VR Signal Expander10/1
  Roll Triangle/1(pts) -> VR Signal Expander4/1
  VR Signal Expander1/1 -> VR Sink1/16, [fg_s]
  Gain5/1 -> Guidance Cross/3(theta)
  If Action Subsystem1/1(Out1) -> Stop Simulation3/1
  VR Signal Expander10/1 -> VR Sink1/18, [at2_t]
  Pitch TranslationText/1(pts) -> VR Signal Expander7/1
  [hdot] -> Vertical Rate/1(hdot)
  [phi] -> Pitch Translation Bars/2(roll)
  [phi] -> Gain4/1
  "Vehicle Dynamics "/24(aE) -> [aE]
  "Vehicle Dynamics "/25(aN) -> [aN]
  Gain12/1 -> Saturation1/1
  Sum7/1 -> Gain12/1
  Sum6/1 -> Gain11/1
  Saturation1/1 -> Switch5/1, To Workspace24/1
  Gain11/1 -> Saturation/1
  [phi] -> Sum6/2
  [thetaG] -> Sum7/1
  [theta] -> Sum7/2
  [phiG] -> Sum6/1
  Data Store Read37/1 -> Switch5/2, Switch2/2
  Saturation/1 -> Switch2/1, To Workspace25/1
  Demux3/8 -> Data Store Write20/1
  AUTO Mode Select1/1(xy) -> VR Signal Expander11/1
  ? -> ?
  Data Store Read39/1 -> AUTO Mode Select1/1(Mode)
  HSI_Ball/1(xy) -> VR Signal Expander12/1, Add1/1
  [VN] -> HSI_Ball/1(VN)
  [VN] -> HSI_Vec/1(VN)
  HSI_Vec/2(scale) -> VR Signal Expander15/1
  [VEG] -> HSI_VG/1(VEG)
  Gain13/1 -> VR Signal Expander33/1
  HSI_LP/2(theta) -> VR Signal Expander16/1
  HSI_Acc1/1(xy) -> Add1/2
  HSI_LP/1(range) -> VR Text Output2/1
  HSI_Vec/1(theta) -> VR Signal Expander14/1
  Constant23/1 -> Switch8/1
  [h] -> Compare To Constant1/1
  [ypos] -> Sum1/2
  [yLP] -> Sum1/1
  Switch8/1 -> Mux3/3
  [ypos] -> Mux3/2
  Compare To Constant1/1 -> Switch8/2
  [xpos] -> Mux3/1
  Add1/1 -> VR Signal Expander32/1
  [VE] -> HSI_Ball/2(VE)
  Mux3/1 -> Gain13/1
  HSI_LP/4(xyHSI) -> VR Signal Expander31/1
  [xpos] -> Sum/2
  [aN] -> HSI_Acc1/2(VNG)
  [VNG] -> HSI_VG/2(VNG)
  HSI_LP/3(xyLP) -> VR Signal Expander17/1
  [aE] -> HSI_Acc1/1(VEG)
  Constant22/1 -> Switch8/3
  [xLP] -> Sum/1
  HSI_VG/1(xy) -> VR Signal Expander30/1
  [VE] -> HSI_Vec/2(VE)
  HSI_Vec/3(xy) -> VR Signal Expander13/1
  IPC Mode Select2/1(xy) -> VR Signal Expander35/1
  AUTO Mode Select3/1(xy) -> VR Signal Expander36/1
  Data Store Read38/1 -> AUTO Mode Select3/1(Mode), IPC Mode Select2/1(Mode), RCAH Mode Select1/1(Mode)
  RCAH Mode Select1/1(xy) -> VR Signal Expander34/1
  Sum/1 -> HSI_LP/1(dLPX)
  Sum1/1 -> HSI_LP/2(dLPY)
  Data Store Read2/1 -> HSD_model/9
  [abort] -> HSD_model/4
  Image From File9/1 -> HSD_model/5
  [ypos] -> HSD_model/8
  Constant2/1 -> HSD_model/1
  [xpos] -> HSD_model/7
  Image From File7/1 -> HSD_model/2
  Image From File8/1 -> HSD_model/3
  [h] -> Compare To Constant/1
  Compare To Constant/1 -> HSD_model/6
  Data Store Read3/1 -> HSD_model/10
  If Action Subsystem6/2(Out2) -> [yLP], Data Store Write22/1
  [h] -> MATLAB Function8/1(h)
  If Action Subsystem6/1(Out1) -> [xLP], Data Store Write6/1
  Constant15/1 -> Switch12/3
  Detect Increase4/1 -> Switch12/2
  MATLAB Function6/1(mode) -> Scope3/1, If5/1, Data Store Write3/1
  [Speed] -> MATLAB Function6/1(speed)
  MATLAB Function8/1(Abort_true) -> If9/2
  Define Buttons LPs1/2(button_IPC) -> Detect Increase4/1, Switch12/1
  If Action Subsystem7/2(Out2) -> [yLP_OG], Switch11/3, If Action Subsystem6/2(yLP)
  Detect Increase1/1 -> Scope2/1, If2/1
  [roll_comm] -> MATLAB Function6/4(roll_com)
  [pitch_comm] -> MATLAB Function6/3(pitch_com)
  [R] -> MATLAB Function6/2(R)
  Define Buttons LPs1/1(button) -> To Workspace10/1, If Action Subsystem7/1(Button)
  Data Store Read6/1 -> If Action Subsystem6/3(Interval)
  Switch12/1 -> To Workspace11/1, If Action Subsystem6/4(button_IPC)
  Delay1/1 -> Stop Simulation4/1
  If9/1 -> If Action Subsystem9/Action
  Joystick Input2/3 -> Terminator6/1
  Joystick Input2/2 -> MATLAB Function6/5(buttons), Define Buttons LPs1/1(buttons), Abort_Value_Func1/1(buttons), Secondary Workload/1(buttons)
  Joystick Input2/1 -> Demux/1
  If2/1 -> If Action Subsystem7/Action
  [fail_detect] -> Secondary Workload/2(fail_detect)
  Secondary Workload/2(fail_button) -> [fail_button]
  Constant11/1 -> MATLAB Function6/6(Avail_Mode)
  Define Buttons LPs1/3(total) -> Detect Increase1/1
  Data Store Read36/1 -> VN output2/1, Switch11/2, Switch7/2
  If Action Subsystem7/1(Out1) -> Switch7/3, [xLP_OG], If Action Subsystem6/1(xLP)
  Abort_Value_Func1/1(Abort) -> If9/1, "  2"/1
  Mux4/1 -> Pitch & Roll1/1
  Detect Change5/1 -> S-R Flip-Flop1/2
  B&E function1/2(fail_time) -> " 2"/1
  Switch10/1 -> ASCII to String1/1
  B&E function1/1(status) -> Detect Change5/1, Switch10/3
  Constant16/1 -> Switch10/1
  [fail_button] -> S-R Flip-Flop1/1
  ASCII to String1/1 -> B&E test1/1
  S-R Flip-Flop1/1 -> Switch10/2
  [phi] -> Mux4/1
  [theta] -> Mux4/2
  [Time] -> B&E function1/1(t)
  MATLAB Function9/2(z_land) -> VR Signal Expander19/1
  MATLAB Function9/1(z_abort) -> VR Signal Expander18/1
  MATLAB Function9/3(z_fuel) -> VR Signal Expander20/1
  [abort] -> MATLAB Function9/3(abort)
  [fuel] -> MATLAB Function9/4(fuel)
  [h] -> MATLAB Function9/1(h)
  Data Store Read18/1 -> MATLAB Function9/2(hLP)
  If Action Subsystem9/1(Out1) -> Delay1/1, "  3"/1, [abort], Scope4/1
  Secondary Workload/1(Detected) -> Scope5/1, " 3"/1
  Switch2/1 -> "Vehicle Dynamics "/1(rollcomm)
  Switch5/1 -> "Vehicle Dynamics "/2("pitchcomm ")
  [R] -> AUTO Mode Select3/2(R)
  Round/1 -> VR Text Output4/1, VR Text Output3/1  "time_to_empty"
  [Speed] -> Round/1
  MATLAB Function14/1(og_lp) -> VR Signal Expander23/1
  Constant1/1 -> MATLAB Function14/3(avail_mode)
  [R] -> AUTO Mode Select1/2(R)
  [xLP_OG] -> Sum4/1
  [xpos] -> Sum4/2
  Sum4/1 -> MATLAB Function14/1(XLP)
  [ypos] -> Sum5/2
  [yLP_OG] -> Sum5/1
  Sum5/1 -> MATLAB Function14/2(YLP)
  VR Signal Expander4/1 -> VR Sink1/1
  VR Signal Expander8/1 -> VR Sink1/2
  VR Signal Expander6/1 -> VR Sink1/7
  VR Signal Expander3/1 -> VR Sink1/10, VR Sink1/14, VR Sink1/6
  VR Signal Expander11/1 -> VR Sink1/13, VR Sink1/9, VR Sink1/8
  VR Signal Expander7/1 -> VR Sink1/11
  VR Signal Expander5/1 -> VR Sink1/12
  VR Signal Expander/1 -> VR Sink1/15
  VR Signal Expander12/1 -> VR Sink/1
  VR Signal Expander14/1 -> VR Sink/2
  VR Signal Expander15/1 -> VR Sink/3
  VR Signal Expander13/1 -> VR Sink/4
  VR Signal Expander16/1 -> VR Sink/5
  VR Signal Expander17/1 -> VR Sink/6
  VR Signal Expander30/1 -> VR Sink/7
  VR Signal Expander31/1 -> VR Sink/8
  VR Signal Expander32/1 -> VR Sink/9
  [fg_s] -> VR Sink/10
  [dl_t] -> VR Sink/11
  [dhtd_t] -> VR Sink/12
  [at_t] -> VR Sink/13
  [at2_t] -> VR Sink/14
  [at1_t] -> VR Sink/15
  VR Signal Expander34/1 -> VR Sink/16
  VR Signal Expander35/1 -> VR Sink/17
  VR Signal Expander36/1 -> VR Sink/18
  VR Signal Expander33/1 -> VR Sink/19
  VR Signal Expander18/1 -> VR Sink/20
  VR Signal Expander19/1 -> VR Sink/21
  VR Signal Expander20/1 -> VR Sink/22
  VR Signal Expander23/1 -> VR Sink/23
  "Vehicle Dynamics "/2(pitch angle) -> pitch output/1, [theta]
  Demux7/16 -> [buzz_time_1]
  Demux7/17 -> [alarm_time_1]
  Demux7/18 -> [buzz_time_2]
  MATLAB Function7/1(ON) -> MATLAB Function/2(tactor)
  MATLAB Function7/3(dur) -> MATLAB Function/4(dur)
  MATLAB Function7/2(Mag) -> MATLAB Function/3(Amp)
  Define Buttons LPs1/5(auditory) -> [auditory_press]
  MATLAB Function15/1(y) -> To Workspace7/1
  [fuel_fail] -> Switch/2
  [fuel] -> To Workspace20/1, If/1
  [fuel_leak] -> "Vehicle Dynamics "/35(In1)
  If Action Subsystem2/1(Out1) -> Merge/1
  If Action Subsystem3/1(Out1) -> Merge/2
  MATLAB Function16/1(out) -> MATLAB Function17/1(u)
  Clock1/1 -> MATLAB Function18/1(time), If1/3, MATLAB Function15/1(time), MATLAB Function16/2(time)
  [auditory_press] -> MATLAB Function18/3(auditory_press)
  Merge/1 -> MATLAB Function16/3(leak), Scope1/1, [fuel_leak]
  From29/1 -> MATLAB Function10/1(time)
  [alarm_time_1] -> MATLAB Function18/2(start_time), If1/2, MATLAB Function16/1(start_time)
  If1/1 -> If Action Subsystem2/Action
  If1/2 -> If Action Subsystem3/Action
  MATLAB Function18/1(out) -> If1/1, [Auditory_press], MATLAB Function15/2(auditory)

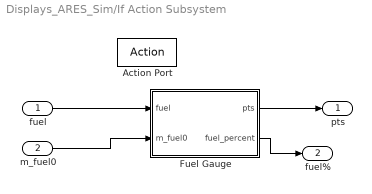
== system Displays_ARES_Sim/If Action Subsystem ==
  fuel : Inport
  m_fuel0 : Inport  Port=2
  Action Port : ActionPort  ActionPortLabel=if(u1 > 0)
  Fuel Gauge : MATLAB Function  TreatAsAtomicUnit=on
  pts : Outport  VectorParamsAs1DForOutWhenUnconnected=off
  fuel% : Outport  Port=2  VectorParamsAs1DForOutWhenUnconnected=off
  wires:
  fuel/1 -> Fuel Gauge/1(fuel)
  Fuel Gauge/1(pts) -> pts/1
  m_fuel0/1 -> Fuel Gauge/2(m_fuel0)
  Fuel Gauge/2(fuel_percent) -> fuel%/1

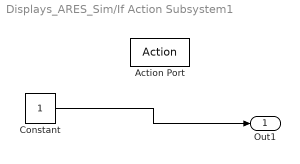
== system Displays_ARES_Sim/If Action Subsystem1 ==
  Action Port : ActionPort  ActionPortLabel=elseif(u1<0)
  Constant : Constant
  Out1 : Outport  InitialOutput=0  VectorParamsAs1DForOutWhenUnconnected=off
  wires:
  Constant/1 -> Out1/1

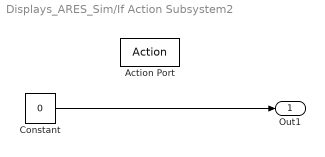
== system Displays_ARES_Sim/If Action Subsystem2 ==
  Action Port : ActionPort  ActionPortLabel=if(u1==1)
  Constant : Constant  Value=0
  Out1 : Outport  InitialOutput=0
  wires:
  Constant/1 -> Out1/1

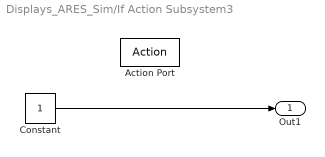
== system Displays_ARES_Sim/If Action Subsystem3 ==
  Action Port : ActionPort  ActionPortLabel=elseif(u2==u3)
  Constant : Constant
  Out1 : Outport  InitialOutput=1
  wires:
  Constant/1 -> Out1/1

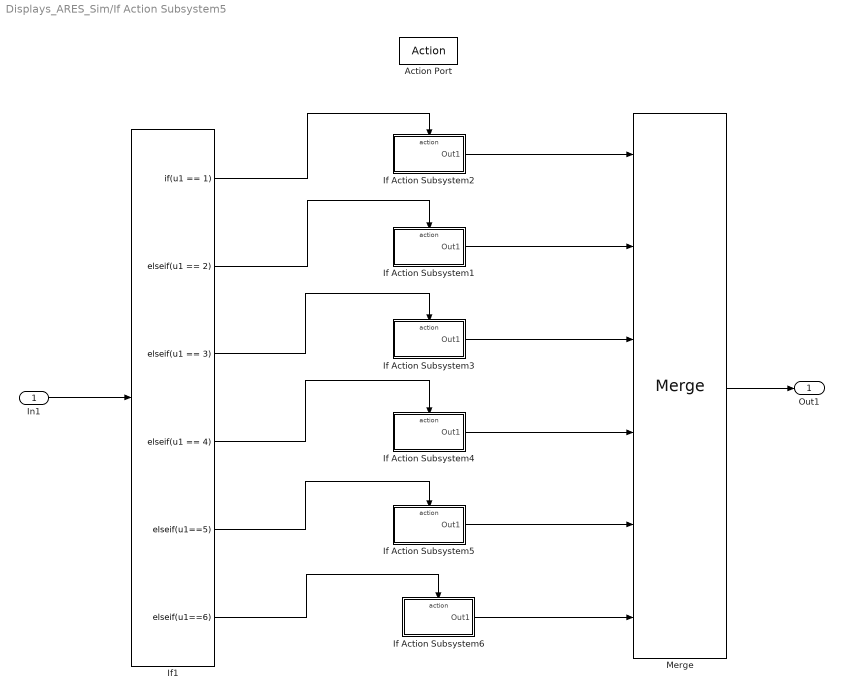
== system Displays_ARES_Sim/If Action Subsystem5 ==
  In1 : Inport
  Action Port : ActionPort  ActionPortLabel=if(u1 > 0)
  If Action Subsystem1 : Subsystem  TreatAsAtomicUnit=on
  If Action Subsystem2 : Subsystem  TreatAsAtomicUnit=on
  If Action Subsystem3 : Subsystem  TreatAsAtomicUnit=on
  If Action Subsystem4 : Subsystem  TreatAsAtomicUnit=on
  If Action Subsystem5 : Subsystem  TreatAsAtomicUnit=on
  If Action Subsystem6 : Subsystem  TreatAsAtomicUnit=on
  If1 : If  IfExpression=u1 == 1  ElseIfExpressions=u1 == 2, u1 == 3, u1 == 4,u1==5,u1==6  ShowElse=off
  Merge : Merge  Inputs=6  InitialOutput=[0;0;0;0;0;0]
  Out1 : Outport  VectorParamsAs1DForOutWhenUnconnected=off
  wires:
  In1/1 -> If1/1
  If1/1 -> If Action Subsystem2/Action
  If1/2 -> If Action Subsystem1/Action
  If1/3 -> If Action Subsystem3/Action
  If1/4 -> If Action Subsystem4/Action
  If Action Subsystem2/1(Out1) -> Merge/1
  If Action Subsystem3/1(Out1) -> Merge/3
  If Action Subsystem4/1(Out1) -> Merge/4
  Merge/1 -> Out1/1
  If Action Subsystem1/1(Out1) -> Merge/2
  If1/5 -> If Action Subsystem5/Action
  If Action Subsystem5/1(Out1) -> Merge/5
  If1/6 -> If Action Subsystem6/Action
  If Action Subsystem6/1(Out1) -> Merge/6

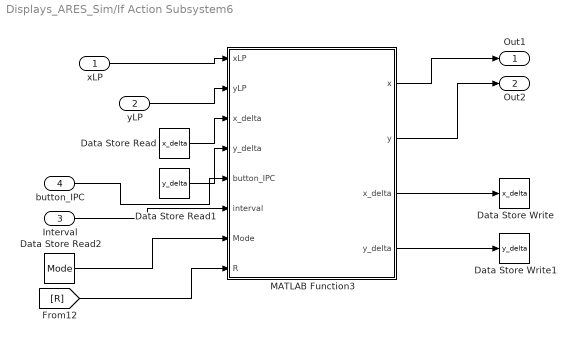
== system Displays_ARES_Sim/If Action Subsystem6 ==
  xLP : Inport
  yLP : Inport  Port=2
  Interval : Inport  Port=3
  button_IPC : Inport  Port=4
  Data Store Read : DataStoreRead  DataStoreName=x_delta
  Data Store Read1 : DataStoreRead  DataStoreName=y_delta
  Data Store Read2 : DataStoreRead  DataStoreName=Mode
  Data Store Write : DataStoreWrite  DataStoreName=x_delta
  Data Store Write1 : DataStoreWrite  DataStoreName=y_delta
  MATLAB Function3 : MATLAB Function  TreatAsAtomicUnit=on
  Out1 : Outport  InitialOutput=[xLP0]  VectorParamsAs1DForOutWhenUnconnected=off
  Out2 : Outport  Port=2  InitialOutput=[yLP0]  VectorParamsAs1DForOutWhenUnconnected=off
  wires:
  MATLAB Function3/1(x) -> Out1/1
  MATLAB Function3/2(y) -> Out2/1
  xLP/1 -> MATLAB Function3/1(xLP)
  yLP/1 -> MATLAB Function3/2(yLP)
  button_IPC/1 -> MATLAB Function3/5(button_IPC)
  Interval/1 -> MATLAB Function3/6(interval)
  Data Store Read/1 -> MATLAB Function3/3("x_delta ")
  MATLAB Function3/3(x_delta) -> Data Store Write/1
  Data Store Read1/1 -> MATLAB Function3/4("y_delta ")
  MATLAB Function3/4(y_delta) -> Data Store Write1/1
  Data Store Read2/1 -> MATLAB Function3/7(Mode)
  [R] -> MATLAB Function3/8(R)
